simulink model "CoolingCheese_Relays"  (R2022a)
settings: Solver=VariableStepAuto  StartTime=0.0  StopTime=H  RelTol=1e-3
values from neighbouring files (symbols this model uses):
  C_c = 2795    [allSimulationParams.mat]
  C_f = 1300    [allSimulationParams.mat]
  k_af = 1.2    [allSimulationParams.mat]
  k_fc = 12    [allSimulationParams.mat]
  q_star = 100    [allSimulationParams.mat]
  theta0_c = 300.31    [allSimulationParams.mat]
  theta0_f = 283.31    [allSimulationParams.mat]
  Ts = 1    [allSimulationParams.mat]
  var_wc = 1    [allSimulationParams.mat]
  var_wf = 1    [allSimulationParams.mat]
settings Model: Creator=mrnel  LastModifiedBy=mrnel

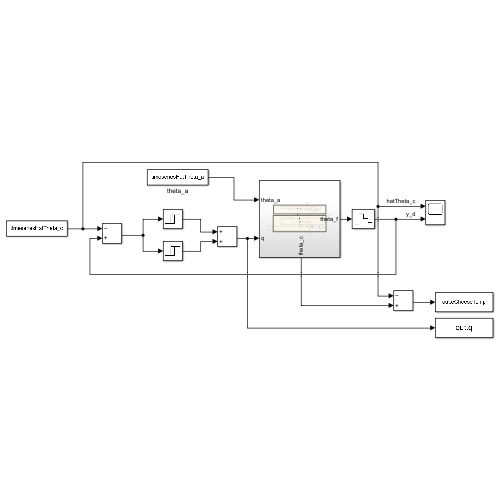
[thumbnail: Simulink's stored preview of the top-level diagram]
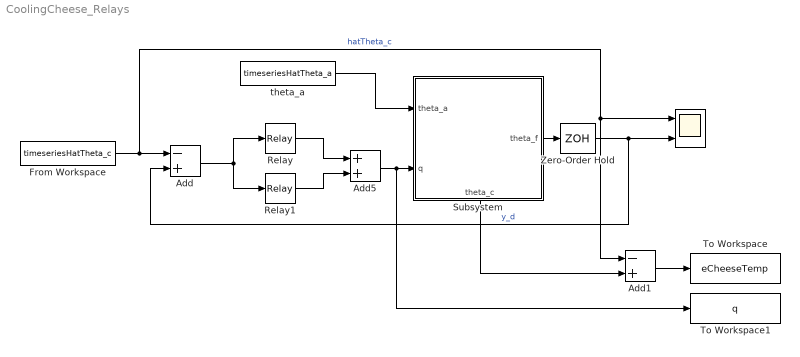
== system CoolingCheese_Relays ==
  " " : Scope  NumInputPorts=2
  Add : Sum  Inputs=-+
  Add1 : Sum  Inputs=-+
  Add5 : Sum
  From Workspace : FromWorkspace  VariableName=timeseriesHatTheta_c  SampleTime=Ts
  Relay : Relay  OnSwitchValue=2  OffSwitchValue=2  OnOutputValue=-q_star/2  OffOutputValue=q_star/2
  Relay1 : Relay  OnSwitchValue=-2  OffSwitchValue=-2  OnOutputValue=-q_star/2  OffOutputValue=q_star/2
  Subsystem : Subsystem
      settings: PortSchema="{\"entries\":[{\"content\":{\"sides\":[{\"content\":{\"connectorIds\":[\"In1\",\"In2\"]},\"type\":\"ConnectorPlacement.EquallySpacedRectSide\",\"uuid\":\"eba34cfc-fb47-492b-95d5-eeb5e4847445\"},{\"content\":{\"connectorIds\":[\"Out1\"],\"side\":\"RIGHT\"},\"type\":\"ConnectorPlacement.EquallySpacedRectSide\",\"uuid\":\"80d274de-5367-4b4d-81b4-04277273f325\"},{\"content\":{\"connectorIds\":[],\"side\":\"TOP\"},\"type\":\"ConnectorPlacement.EquallySpacedRectSide\",\"uuid\":\"43daf5e6-3a1e-44cb-a044-8143443f2aa6\"},{\"content\":{\"connectorIds\":[\"Out2\"],\"side\":\"BOTTOM\"},\"type\":\"ConnectorPlacement.EquallySpacedRectSide\",\"uuid\":\"e46d0b73-af70-4fc9-81e4-f7db7a36aa9f\"}]},\"type\":\"ConnectorPlacement.EquallySpacedConnector\",\"uuid\":\"5e0d6d6e-93f8-4b3e-b8a3-23aa4f63c8e1\"}],\"packageUris\":[\"http://schema.mathworks.com/mf0/Connector/R2020b\"],\"version\":\"1.0\"}"
  To Workspace : ToWorkspace  VariableName=eCheeseTemp  SaveFormat=Timeseries  SampleTime=Ts
  To Workspace1 : ToWorkspace  VariableName=q  SaveFormat=Timeseries  SampleTime=Ts
  Zero-Order Hold : ZeroOrderHold  SampleTime=Ts
  theta_a : FromWorkspace  VariableName=timeseriesHatTheta_a  SampleTime=Ts
  wires:
  theta_a/1 -> Subsystem/1(theta_a)
  Subsystem/1(theta_f) -> Zero-Order Hold/1
  Zero-Order Hold/1 -> Add/2, " "/2  "y_d"
  Relay/1 -> Add5/1
  Relay1/1 -> Add5/2
  Add/1 -> Relay1/1, Relay/1
  Add1/1 -> To Workspace/1
  Subsystem/2(theta_c) -> Add1/2
  From Workspace/1 -> Add1/1, " "/1, Add/1  "hatTheta_c"
  Add5/1 -> To Workspace1/1, Subsystem/2(q)

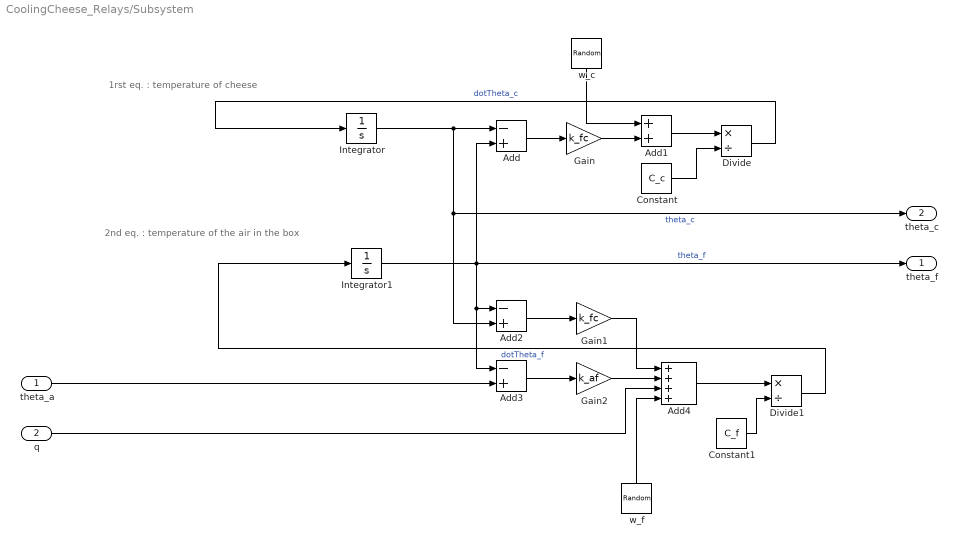
== system CoolingCheese_Relays/Subsystem ==
  note: 2nd eq. : temperature of the air in the box
  note: 1rst eq. : temperature of cheese
  theta_a : Inport
  q : Inport  Port=2
  Add : Sum  Inputs=-+
  Add1 : Sum
  Add2 : Sum  Inputs=-+
  Add3 : Sum  Inputs=-+
  Add4 : Sum  Inputs=++++
  Constant : Constant  Value=C_c
  Constant1 : Constant  Value=C_f
  Divide : Product  Inputs=*/
  Divide1 : Product  Inputs=*/
  Gain : Gain  Gain=k_fc
  Gain1 : Gain  Gain=k_fc
  Gain2 : Gain  Gain=k_af
  Integrator : Integrator  InitialCondition=theta0_c
  Integrator1 : Integrator  InitialCondition=theta0_f
  w_c : RandomNumber  Variance=var_wc  SampleTime=Ts
  w_f : RandomNumber  Variance=var_wf  SampleTime=Ts
  theta_f : Outport
  theta_c : Outport  Port=2
  wires:
  Gain2/1 -> Add4/2
  Divide/1 -> Integrator/1  "dotTheta_c"
  Add2/1 -> Gain1/1
  Add1/1 -> Divide/1
  Divide1/1 -> Integrator1/1  "dotTheta_f"
  w_c/1 -> Add1/1
  Integrator/1 -> Add2/2, theta_c/1, Add/1  "theta_c"
  Integrator1/1 -> theta_f/1, Add3/1, Add2/1, Add/2  "theta_f"
  Gain/1 -> Add1/2
  Add/1 -> Gain/1
  Constant1/1 -> Divide1/2
  w_f/1 -> Add4/4
  Constant/1 -> Divide/2
  Gain1/1 -> Add4/1
  Add3/1 -> Gain2/1
  Add4/1 -> Divide1/1
  q/1 -> Add4/3
  theta_a/1 -> Add3/2
